simulink model "HW"  (R2022b)
settings: Solver=VariableStepAuto  StartTime=0.0  StopTime=10.0  FixedStep=0.0001  MaxStep=0.001  RelTol=1e-3
values from neighbouring files (symbols this model uses):
  a_sin = [pi/2; pi/2; 0.2; pi/2]    [HW_par.m]
  Kd = 1000*eye(4)    [HW_par.m]
  Kp = 1000*eye(4)    [HW_par.m]
  omega_sin = 10*[1; 1; 1; 1]    [HW_par.m]
  q_0 = [0;0;0;0]    [HW_par.m]
  q_dot_0 = [0;0;0;0]    [HW_par.m]
  q_target = [pi/2; pi/3; 0.1; -pi/4]    [HW_par.m]
undefined symbols (not defined in the file or in its folder): a_filt, b_filt
settings Model: Creator=Alberto  LastModifiedBy=Christian Russo
settings SolverCC: AlgebraicLoopSolver=TrustRegion
settings DebuggingCC: UnconnectedInputMsg=warning  UnconnectedOutputMsg=warning  UnconnectedLineMsg=warning  SFMachineParentedDataDiag=warning
settings ModelReferenceCC: EnableRefExpFcnMdlSchedulingChecks=on
settings RTWCC: DLArmComputeVersion=19.05

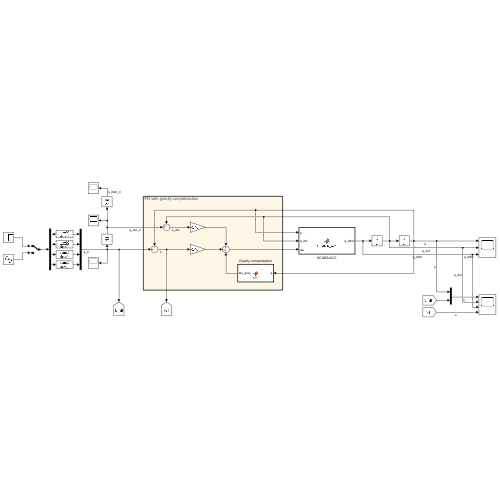
[thumbnail: Simulink's stored preview of the top-level diagram]
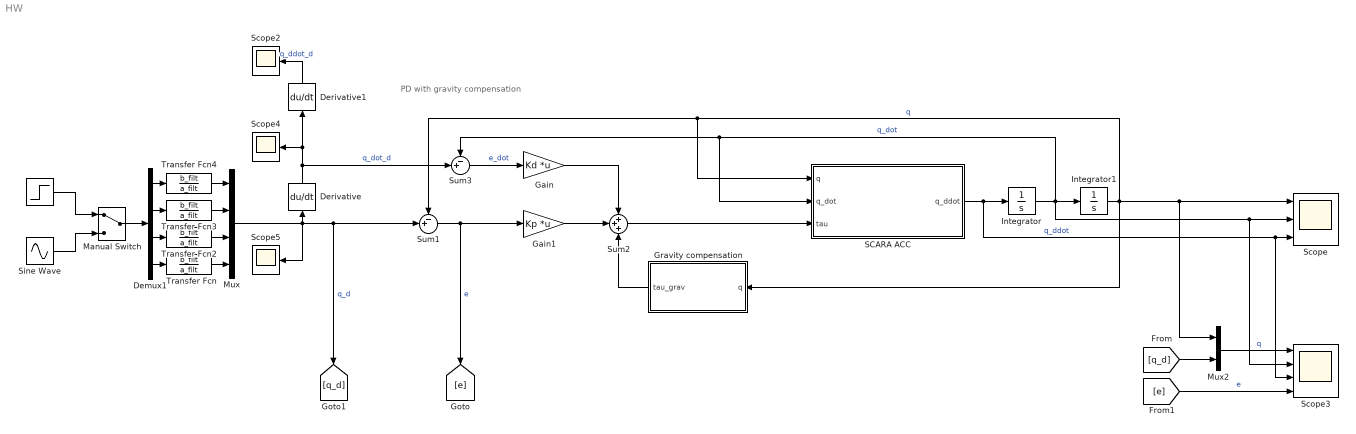
== system HW ==
  note: PD with gravity compensation
  " " : Step  After=q_target  SampleTime=0
  Demux1 : Demux
  Derivative : Derivative
  Derivative1 : Derivative
  Gain : Gain  Gain=Kd  Multiplication=Matrix(K*u)
  Gain1 : Gain  Gain=Kp  Multiplication=Matrix(K*u)
  Gravity compensation : MATLAB Function  TreatAsAtomicUnit=on
  Integrator : Integrator  InitialCondition=q_dot_0
  Integrator1 : Integrator  InitialCondition=q_0
  Manual Switch : ManualSwitch
  Mux : Mux
  Mux2 : Mux  Inputs=2
  SCARA ACC : MATLAB Function  TreatAsAtomicUnit=on
  Scope : Scope  NumInputPorts=3
  Scope2 : Scope
  Scope3 : Scope  NumInputPorts=4
  Scope4 : Scope
  Scope5 : Scope
  Sine Wave : Sin  Amplitude=a_sin  Frequency=omega_sin  SampleTime=0
  Sum1 : Sum  Inputs=-+|
  Sum2 : Sum  Inputs=+++
  Sum3 : Sum  Inputs=-+|
  Transfer Fcn{,2..4} (4 alike) : TransferFcn  Numerator=b_filt  Denominator=a_filt
  wires:
  SCARA ACC/1(q_ddot) -> Integrator/1, Scope3/3, Scope/3  "q_ddot"
  Demux1/1 -> Transfer Fcn4/1
  Demux1/2 -> Transfer Fcn3/1
  Demux1/3 -> Transfer Fcn2/1
  Demux1/4 -> Transfer Fcn/1
  Transfer Fcn4/1 -> Mux/1
  Transfer Fcn3/1 -> Mux/2
  Transfer Fcn2/1 -> Mux/3
  Transfer Fcn/1 -> Mux/4
  Mux/1 -> Sum1/2, [q_d], Scope5/1, Derivative/1  "q_d"
  Manual Switch/1 -> Demux1/1
  " "/1 -> Manual Switch/1
  Sine Wave/1 -> Manual Switch/2
  Derivative/1 -> Sum3/2, Derivative1/1, Scope4/1  "q_dot_d"
  Derivative1/1 -> Scope2/1  "q_ddot_d"
  Sum3/1 -> Gain/1  "e_dot"
  Sum1/1 -> Gain1/1, [e]  "e"
  Gravity compensation/1(tau_grav) -> Sum2/3
  Sum2/1 -> SCARA ACC/3(tau)
  Gain1/1 -> Sum2/2
  Gain/1 -> Sum2/1
  Mux2/1 -> Scope3/1  "q"
  [q_d] -> Mux2/2
  Integrator/1 -> SCARA ACC/2(q_dot), Sum3/1, Integrator1/1, Scope3/2, Scope/2  "q_dot"
  [e] -> Scope3/4  "e"
  Integrator1/1 -> Gravity compensation/1(q), SCARA ACC/1(q), Sum1/1, Mux2/1, Scope/1  "q"

== matlab function HW/SCARA ACC ==
  data: q input; q_ddot output; q_dot input; tau input
function q_ddot = SCARA_acc(q, q_dot, tau)%#codegen
coder.extrinsic('f_B_mex'); 
coder.extrinsic('f_C_vect_mex'); 
coder.extrinsic('f_g_vect_mex');
B = eye(4);
C_vect = zeros(4,1);
F_g = zeros(4,1);
tau = reshape(tau,4,1);
q_ddot = zeros(4,1);
B = full(f_B_mex('f_B',q));
C_vect = full(f_C_vect_mex('f_C_vect', q, q_dot));
F_g = full(f_g_vect_mex('f_g_vect', q));
q_ddot = (eye(4)/B)*(-C_vect-F_g+tau);

== matlab function HW/Gravity compensation ==
  data: q input; tau_grav output
function tau_grav = fcn(q)%#codegen
coder.extrinsic('f_g_vect_mex');
tau_grav = zeros(4,1);
tau_grav = reshape(full(f_g_vect_mex('f_g_vect', q)),4,1);
